simulink library "IP"  (R2014b)
settings: Solver=ode45  StartTime=0.0  StopTime=10.0  RelTol=1e-3
undefined symbols (not defined in the file or in its folder): Serial_Port, Standard_Devices
libraries: IP x7, rtwinlib x4, simulink x2
settings Model: Creator=ZRazer  LastModifiedBy=gt60

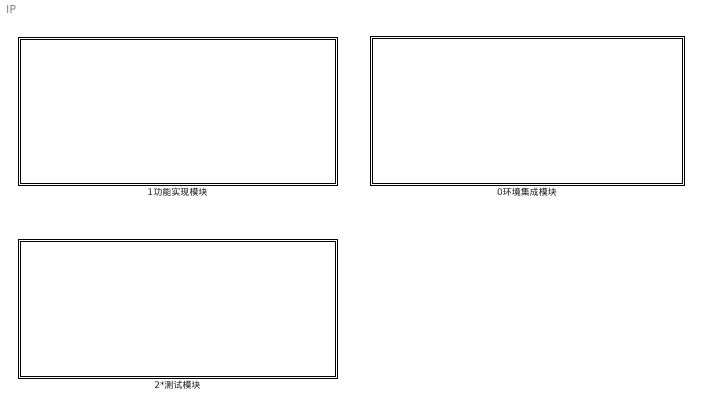
== system IP ==
  0环境集成模块 : Subsystem
  1功能实现模块 : Subsystem
  2*测试模块 : Subsystem

== system IP/0环境集成模块 ==
  倒立摆集成实验 : Subsystem  Description=采样时间dt=0.002s  mask{t=0.002}
      mask prompts: t "sample time(非负数)"
      settings: AttributesFormatString=%<Description>  CopyFcn=set_param(gcbh,'LinkStatus','none');
      mask DialogControl Container5 Prompt: 系统设置
      mask DialogControl ParameterGroupVar Prompt: 采样时间
      mask Display: disp('倒立摆集成模块')
  环境集成实验 : Subsystem  Description=采样时间dt=0.002s  mask{t=0.002}
      mask prompts: t "sample time(非负数)"
      settings: AttributesFormatString=%<Description>  CopyFcn=set_param(gcbh,'LinkStatus','none');
      mask DialogControl Container5 Prompt: 系统设置
      mask DialogControl ParameterGroupVar Prompt: 采样时间
      mask Display: disp('集成环境模块')

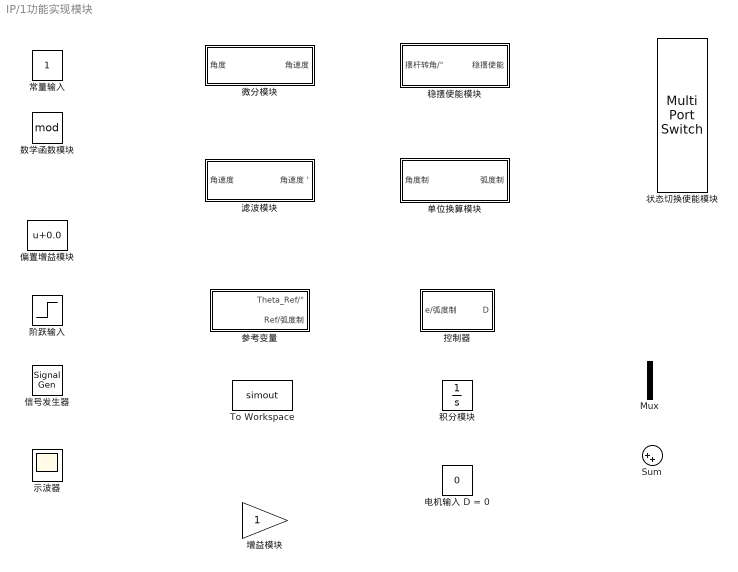
== system IP/1功能实现模块 ==
  Mux : Mux  Inputs=2
  Sum : Sum  Inputs=|++
  To Workspace : ToWorkspace  VariableName=simout  SaveFormat=Timeseries  SampleTime=-1
      settings: AttributesFormatString=%<Description>
      settings: Description=|
      | 数据输出模块
      | 运行完毕后可将连接信号线数据输出到MatLab的工作空间，调用plot命令即可完成数据可视化
      | 调用格式plot(变量名.time，变量名.signals.values)
      | 如：变量名称为theta，在MatLab中调用命令plot(theta.time,theta.signals.values)
  信号发生器 : SignalGenerator  Units=rad/sec
  偏置增益模块 : Bias  Bias=0.0
  单位换算模块 : Subsystem  Description=|
      | 输入：转角(°)或转速(°/s)
      | 输出：转角(rad)或转速(rad/°)
      settings: AttributesFormatString=%<Description>
      mask DialogControl DescGroupVar Prompt: 描述
      mask DialogControl DescTextVar Prompt: 角度制转弧度制
  参考变量 : Subsystem  mask{Amplitude=40, T=10}
      mask prompts: Amplitude "幅值Amplitude/°"; T "周期T/s"
      mask DialogControl Control1 Prompt: 变量期望值
  "增益模块 " : Gain
  常量输入 : Constant
  微分模块 : Subsystem  Description=|
      | 描述：离散微分模块
      | 该部分不必修改
      settings: AttributesFormatString=%<Description>
      mask DialogControl DescGroupVar Prompt: 描述
      mask DialogControl DescTextVar Prompt: 角度-角速度转换
  控制器 : Subsystem  mask{K=[0.0500   0.0258   0.4535   0.0387]}
  数学函数模块 : Math  Description=|  Operator=mod  SaturateOnIntegerOverflow=on
      | 描述：数学函数模块
      | mod 求余函数
      settings: AttributesFormatString=%<Description>
  滤波模块 : Subsystem  Description=|  mask{num=[1], den=[1 2]}
      | 描述：离散滤波模块
      | 先在matlab内构建滤波器的连续传递函数
      | 再内调用c2d()函数
      settings: AttributesFormatString=%<Description>
  状态切换使能模块 : MultiPortSwitch  Description=|  DataPortOrder=Zero-based contiguous  Inputs=2  zeroidx=on
      | 定义左侧端口从上到下分别为输入1~3
      | 输入1：连接稳摆使能端口
      | 输入2：连接常量D=0端口
      | 输入3：连接稳摆控制端口
      | 定义右侧端口为输出端口
      | 输出1：连接控制输入端口
      settings: AttributesFormatString=%<Description>
  "电机输入 D = 0 " : Constant  Description=该模块为输入为0的常量，无法修改  Value=0
      settings: AttributesFormatString=%<Description>
      mask DialogControl DescGroupVar Prompt: 非稳摆状态输入设置
      mask DialogControl DescTextVar Prompt: 控制量u = 0
  示波器 : Scope
      settings: SampleInput=on
  积分模块 : Integrator
  稳摆使能模块 : Subsystem  Description=|  mask{Deg=15}
      | 输入单位：度/°
      | 输出：      0或1
      | 若转角在该范围内，输出1
      | 若转角不在范围内，输出0
      settings: AttributesFormatString=%<Description>
  阶跃输入 : Step  SampleTime=0

== system IP/2*测试模块 ==
  测试模块 : Subsystem  mask{Parameter1=0}

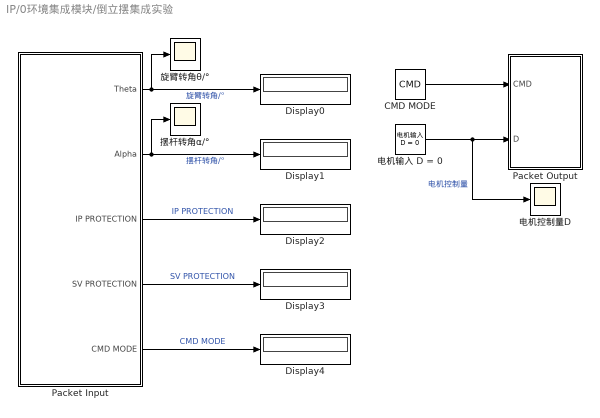
== system IP/0环境集成模块/倒立摆集成实验 ==
  CMD MODE : Constant  Value=CMD  mask{CMD=0}
      mask prompts: CMD "模式选择"
      mask DialogControl DescGroupVar Prompt: 模式切换输入端
      mask DialogControl DescTextVar_copy_copy_copy Prompt: 1:倒立摆模式
      mask DialogControl DescTextVar_copy_copy_copy_copy Prompt: 2:倒立摆异常清除
  Display{0..4} (5 alike) : Display
  Packet Input : Subsystem
  Packet Output : Subsystem
  摆杆转角α/° : Scope
      settings: ShowLegends=on  YMin=-60  YMax=60  SaveName=alpha
  旋臂转角θ/° : Scope
      settings: ShowLegends=on  YMin=-60  YMax=60  SaveName=theta1
  电机控制量D : Scope
      settings: ShowLegends=on  YMin=-0.8  YMax=0.6  SaveName=D
  "电机输入 D = 0 " : IP/附加模块/电机输入 D = 0 
  wires:
  Packet Input/2(Alpha) -> 摆杆转角α/°/1, Display1/1  "摆杆转角/°"
  CMD MODE/1 -> Packet Output/1(CMD)
  Packet Input/1(Theta) -> Display0/1, 旋臂转角θ/°/1  "旋臂转角/°"
  Packet Input/3(IP PROTECTION) -> Display2/1  "IP PROTECTION"
  Packet Input/4(SV PROTECTION) -> Display3/1  "SV PROTECTION"
  Packet Input/5(CMD MODE) -> Display4/1  "CMD MODE"
  "电机输入 D = 0 "/1 -> Packet Output/2(D), 电机控制量D/1  "电机控制量"

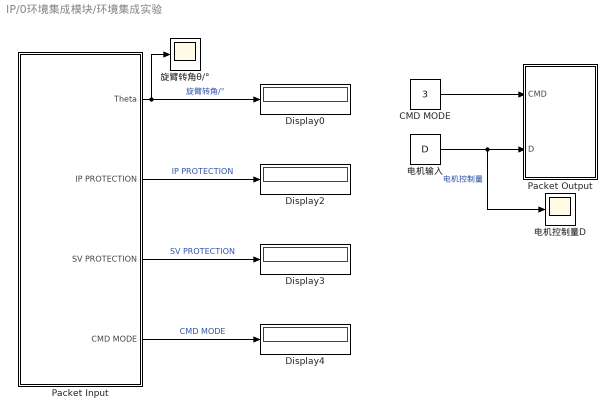
== system IP/0环境集成模块/环境集成实验 ==
  CMD MODE : Constant  Value=3
      mask DialogControl DescGroupVar Prompt: 模式切换输入端
      mask DialogControl DescTextVar Prompt: 当前工作模式：伺服模式(MODE 3）
  Display{0,2..4} (4 alike) : Display
  Packet Input : Subsystem
  Packet Output : Subsystem
  旋臂转角θ/° : Scope
      settings: ShowLegends=on  YMin=-60  YMax=60  SaveName=theta
  电机控制量D : Scope
      settings: ShowLegends=on  YMin=-0.8  YMax=0.6  SaveName=D1
  电机输入 : Constant  Value=D  mask{D=0.0}
      mask DialogControl DescGroupVar Prompt: 电机输入
      mask DialogControl DescTextVar Prompt: 占空比大小
  wires:
  CMD MODE/1 -> Packet Output/1(CMD)
  Packet Input/1(Theta) -> 旋臂转角θ/°/1, Display0/1  "旋臂转角/°"
  Packet Input/2(IP PROTECTION) -> Display2/1  "IP PROTECTION"
  Packet Input/3(SV PROTECTION) -> Display3/1  "SV PROTECTION"
  Packet Input/4(CMD MODE) -> Display4/1  "CMD MODE"
  电机输入/1 -> Packet Output/2(D), 电机控制量D/1  "电机控制量"

== system IP/1功能实现模块/单位换算模块 ==
  角度制 : Inport
  Deg2Rad : Gain  Gain=pi/180
  弧度制 : Outport
  wires:
  角度制/1 -> Deg2Rad/1
  Deg2Rad/1 -> 弧度制/1

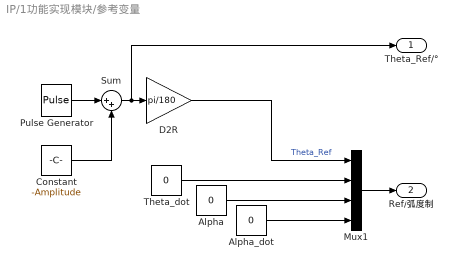
== system IP/1功能实现模块/参考变量 ==
  Alpha : Constant  Value=0
  Alpha_dot : Constant  Value=0
  Constant : Constant  Value=-Amplitude  SampleTime=-1
  D2R : Gain  Gain=pi/180
  Mux1 : Mux
  Pulse Generator : DiscretePulseGenerator  PulseType=Time based  Amplitude=Amplitude*2  Period=T  PulseWidth=50
  Sum : Sum  Inputs=|++
  "Theta_dot " : Constant  Value=0
  Theta_Ref/° : Outport
  Ref/弧度制 : Outport  Port=2
  wires:
  Pulse Generator/1 -> Sum/1
  Constant/1 -> Sum/2
  Sum/1 -> Theta_Ref/°/1, D2R/1
  "Theta_dot "/1 -> Mux1/2
  Alpha_dot/1 -> Mux1/4
  Mux1/1 -> Ref/弧度制/1
  Alpha/1 -> Mux1/3
  D2R/1 -> Mux1/1  "Theta_Ref"

== system IP/1功能实现模块/微分模块 ==
  角度 : Inport
  Difference : simulink/Discrete/Difference  ICPrevInput=0.0  InputProcessing=Inherited  OutMin=[]  OutMax=[]  OutDataType=fixdt(1, 16)  OutScaling=2^-10  DoSatur=off
  补偿1/t : Gain  Gain=1/t
  角速度 : Outport
  wires:
  角度/1 -> Difference/1
  补偿1/t/1 -> 角速度/1
  Difference/1 -> 补偿1/t/1

== system IP/1功能实现模块/控制器 ==
  e/弧度制 : Inport
  Gain : Gain  Gain=K  Multiplication=Matrix(K*u)
  Gain1 : Gain  Gain=-1
  D : Outport
  wires:
  e/弧度制/1 -> Gain/1
  Gain/1 -> Gain1/1
  Gain1/1 -> D/1

== system IP/1功能实现模块/滤波模块 ==
  角速度 : Inport
  Discrete Transfer Fcn1 : DiscreteTransferFcn  Numerator=num  Denominator=den
  角速度 ' : Outport
  wires:
  Discrete Transfer Fcn1/1 -> 角速度 '/1
  角速度/1 -> Discrete Transfer Fcn1/1

== system IP/1功能实现模块/稳摆使能模块 ==
  摆杆转角/° : Inport
  Enable : simulink/Logic and Bit Operations/Compare To Constant  relop=<=  const=Deg  OutDataTypeStr=uint8  ZeroCross=off
  |Alpha_Balance| : Abs
  稳摆使能 : Outport
  wires:
  摆杆转角/°/1 -> |Alpha_Balance|/1
  Enable/1 -> 稳摆使能/1
  |Alpha_Balance|/1 -> Enable/1

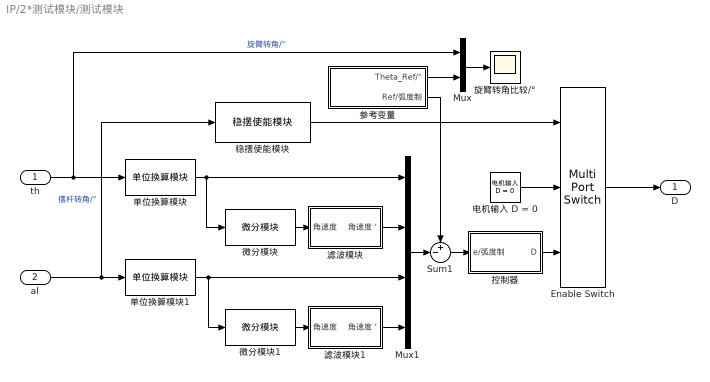
== system IP/2*测试模块/测试模块 ==
  th : Inport
  al : Inport  Port=2
  Enable Switch : MultiPortSwitch  DataPortOrder=Zero-based contiguous  Inputs=2  zeroidx=on
  Mux : Mux  Inputs=2
  Mux1 : Mux
  Sum1 : Sum  Inputs=+-|
  单位换算模块 : IP/附加模块/单位换算模块
      settings: AttributesFormatString=%<Description>
  单位换算模块1 : IP/附加模块/单位换算模块
      settings: AttributesFormatString=%<Description>
  参考变量 : Subsystem  mask{Amplitude=40, T=10}
      mask prompts: Amplitude "幅值Amplitude/°"; T "周期T/s"
      mask DialogControl Control1 Prompt: 变量期望值
  微分模块 : IP/附加模块/微分模块
      settings: AttributesFormatString=%<Description>
  微分模块1 : IP/附加模块/微分模块
      settings: AttributesFormatString=%<Description>
  控制器 : Subsystem  mask{K=[0.0500   0.0258   0.4535   0.0387]}
  旋臂转角比较/° : Scope
      settings: ShowLegends=on  YMin=-80  YMax=80  SaveName=cmp
  滤波模块 : Subsystem  mask{num=[0.2212], den=[1 -0.7788]}
      settings: AttributesFormatString=%<Description>
  滤波模块1 : Subsystem  mask{num=[0.2212], den=[1 -0.7788]}
      settings: AttributesFormatString=%<Description>
  "电机输入 D = 0 " : IP/附加模块/电机输入 D = 0 
  稳摆使能模块 : IP/附加模块/稳摆使能模块  Deg=15
      settings: AttributesFormatString=%<Description>
  D : Outport
  wires:
  al/1 -> 稳摆使能模块/1, 单位换算模块1/1  "摆杆转角/°"
  th/1 -> Mux/1, 单位换算模块/1  "旋臂转角/°"
  "电机输入 D = 0 "/1 -> Enable Switch/2
  稳摆使能模块/1 -> Enable Switch/1
  单位换算模块1/1 -> 微分模块1/1, Mux1/3
  微分模块/1 -> 滤波模块/1(角速度)
  微分模块1/1 -> 滤波模块1/1(角速度)
  滤波模块/1(角速度 ') -> Mux1/2
  滤波模块1/1(角速度 ') -> Mux1/4
  参考变量/1(Theta_Ref/°) -> Mux/2
  Mux/1 -> 旋臂转角比较/°/1
  单位换算模块/1 -> 微分模块/1, Mux1/1
  Sum1/1 -> 控制器/1(e/弧度制)
  Mux1/1 -> Sum1/2
  参考变量/2(Ref/弧度制) -> Sum1/1
  控制器/1(D) -> Enable Switch/3
  Enable Switch/1 -> D/1

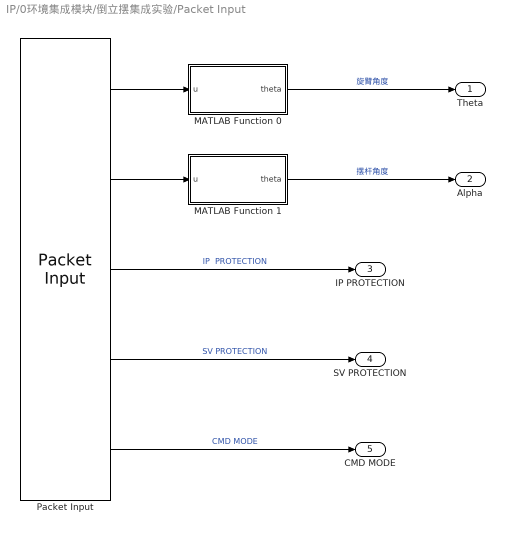
== system IP/0环境集成模块/倒立摆集成实验/Packet Input ==
  MATLAB Function 0 : MATLAB Function  TreatAsAtomicUnit=on
  MATLAB Function 1 : MATLAB Function  TreatAsAtomicUnit=on
  Packet Input : rtwinlib/Packet Input  SampleTime=t  MaxMissedTicks=10  ShowMissedTicks=off  YieldWhenWaiting=off  DrvName=Standard_Devices/Serial_Port  DrvAddress=3  DrvOptions=[460800 8 0 0 0 0 0 0]  PacketSize=9  DataTypes={'int32','int16','uint8','uint8','uint8'}  ShowReady=off  ShowError=off  PacketID=1  ByteOrder=1  ShowTimestamp=off
      settings: AttributesFormatString=Standard Devices\nSerial Port [3h]
  Theta : Outport
  Alpha : Outport  Port=2
  IP PROTECTION : Outport  Port=3
  SV PROTECTION : Outport  Port=4
  CMD MODE : Outport  Port=5
  wires:
  MATLAB Function 1/1(theta) -> Alpha/1  "摆杆角度"
  Packet Input/5 -> CMD MODE/1  "CMD MODE"
  Packet Input/3 -> IP PROTECTION/1  "IP  PROTECTION"
  Packet Input/4 -> SV PROTECTION/1  "SV PROTECTION"
  Packet Input/2 -> MATLAB Function 1/1(u)
  Packet Input/1 -> MATLAB Function 0/1(u)
  MATLAB Function 0/1(theta) -> Theta/1  "旋臂角度"

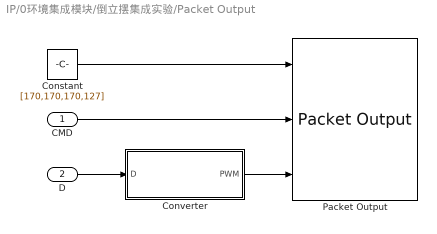
== system IP/0环境集成模块/倒立摆集成实验/Packet Output ==
  CMD : Inport
  D : Inport  Port=2
  Constant : Constant  Value=[170,170,170,127]
      mask DialogControl DescGroupVar Prompt: 描述
      mask DialogControl DescTextVar Prompt: 常量
  Converter : Subsystem  mask{k=0.3}
      mask DialogControl DescTextVar Prompt: 数学变换
  Packet Output : rtwinlib/Packet Output  SampleTime=t  MaxMissedTicks=10  ShowMissedTicks=off  YieldWhenWaiting=off  DrvName=Standard_Devices/Serial_Port  DrvAddress=3  DrvOptions=[460800 8 0 0 0 0 0 0]  PacketSize=7  DataTypes={'4*uint8','uint8','int16'}  ShowReady=off  ShowError=off  PacketID=1  ByteOrder=1  InitialValue=[170 170 170 127 1 0]  FinalValue=[]
      settings: AttributesFormatString=Standard Devices\nSerial Port [3h]
  wires:
  D/1 -> Converter/1(D)
  Constant/1 -> Packet Output/1
  Converter/1(PWM) -> Packet Output/3
  CMD/1 -> Packet Output/2

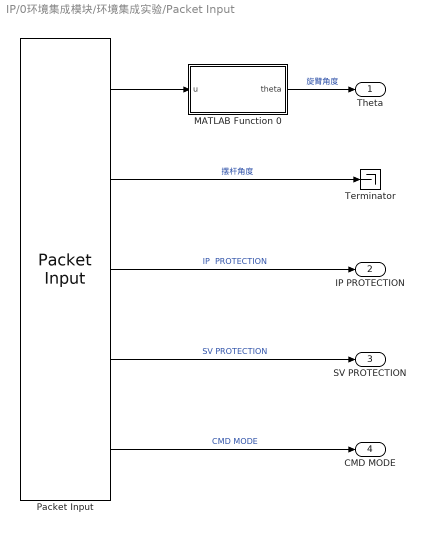
== system IP/0环境集成模块/环境集成实验/Packet Input ==
  MATLAB Function 0 : MATLAB Function  TreatAsAtomicUnit=on
  Packet Input : rtwinlib/Packet Input  SampleTime=t  MaxMissedTicks=10  ShowMissedTicks=off  YieldWhenWaiting=off  DrvName=Standard_Devices/Serial_Port  DrvAddress=3  DrvOptions=[460800 8 0 0 0 0 0 0]  PacketSize=9  DataTypes={'int32','int16','uint8','uint8','uint8'}  ShowReady=off  ShowError=off  PacketID=1  ByteOrder=1  ShowTimestamp=off
      settings: AttributesFormatString=Standard Devices\nSerial Port [3h]
  Terminator : Terminator
  Theta : Outport
  IP PROTECTION : Outport  Port=2
  SV PROTECTION : Outport  Port=3
  CMD MODE : Outport  Port=4
  wires:
  Packet Input/2 -> Terminator/1  "摆杆角度"
  Packet Input/5 -> CMD MODE/1  "CMD MODE"
  Packet Input/3 -> IP PROTECTION/1  "IP  PROTECTION"
  Packet Input/4 -> SV PROTECTION/1  "SV PROTECTION"
  Packet Input/1 -> MATLAB Function 0/1(u)
  MATLAB Function 0/1(theta) -> Theta/1  "旋臂角度"

== system IP/0环境集成模块/环境集成实验/Packet Output ==
  CMD : Inport
  D : Inport  Port=2
  Constant : Constant  Value=[170,170,170,127]
      mask DialogControl DescGroupVar Prompt: 描述
      mask DialogControl DescTextVar Prompt: 常量
  Converter : Subsystem  mask{k=0.3}
      mask DialogControl DescTextVar Prompt: 数学变换
  Packet Output : rtwinlib/Packet Output  SampleTime=t  MaxMissedTicks=10  ShowMissedTicks=off  YieldWhenWaiting=off  DrvName=Standard_Devices/Serial_Port  DrvAddress=3  DrvOptions=[460800 8 0 0 0 0 0 0]  PacketSize=7  DataTypes={'4*uint8','uint8','int16'}  ShowReady=off  ShowError=off  PacketID=1  ByteOrder=1  InitialValue=[170 170 170 127 1 0]  FinalValue=[]
      settings: AttributesFormatString=Standard Devices\nSerial Port [3h]
  wires:
  CMD/1 -> Packet Output/2
  Converter/1(PWM) -> Packet Output/3
  Constant/1 -> Packet Output/1
  D/1 -> Converter/1(D)

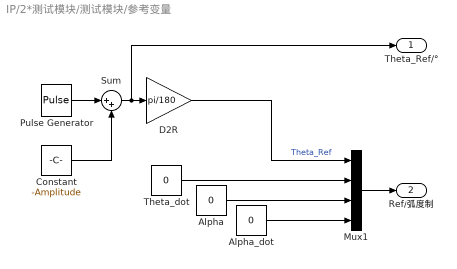
== system IP/2*测试模块/测试模块/参考变量 ==
  Alpha : Constant  Value=0
  Alpha_dot : Constant  Value=0
  Constant : Constant  Value=-Amplitude
  D2R : Gain  Gain=pi/180
  Mux1 : Mux
  Pulse Generator : DiscretePulseGenerator  PulseType=Time based  Amplitude=Amplitude*2  Period=T  PulseWidth=50
  Sum : Sum  Inputs=|++
  "Theta_dot " : Constant  Value=0
  Theta_Ref/° : Outport
  Ref/弧度制 : Outport  Port=2
  wires:
  Pulse Generator/1 -> Sum/1
  Constant/1 -> Sum/2
  Sum/1 -> Theta_Ref/°/1, D2R/1
  "Theta_dot "/1 -> Mux1/2
  Alpha_dot/1 -> Mux1/4
  Mux1/1 -> Ref/弧度制/1
  Alpha/1 -> Mux1/3
  D2R/1 -> Mux1/1  "Theta_Ref"

== system IP/2*测试模块/测试模块/控制器 ==
  e/弧度制 : Inport
  Gain : Gain  Gain=K  Multiplication=Matrix(K*u)
  Gain1 : Gain  Gain=-1
  D : Outport
  wires:
  e/弧度制/1 -> Gain/1
  Gain/1 -> Gain1/1
  Gain1/1 -> D/1

== system IP/2*测试模块/测试模块/滤波模块 ==
  角速度 : Inport
  Discrete Transfer Fcn1 : DiscreteTransferFcn  Numerator=num  Denominator=den
  角速度 ' : Outport
  wires:
  角速度/1 -> Discrete Transfer Fcn1/1
  Discrete Transfer Fcn1/1 -> 角速度 '/1

== system IP/2*测试模块/测试模块/滤波模块1 ==
  角速度 : Inport
  Discrete Transfer Fcn1 : DiscreteTransferFcn  Numerator=num  Denominator=den
  角速度 ' : Outport
  wires:
  Discrete Transfer Fcn1/1 -> 角速度 '/1
  角速度/1 -> Discrete Transfer Fcn1/1

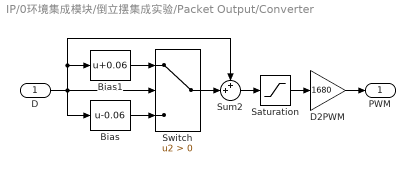
== system IP/0环境集成模块/倒立摆集成实验/Packet Output/Converter ==
  D : Inport
  Bias : Bias  Bias=-0.06
  Bias1 : Bias  Bias=0.06
  D2PWM : Gain  Gain=1680
      mask DialogControl Container4 Prompt: 描述
      mask DialogControl DescTextVar Prompt: 输入占空比-输入PWM
  Saturation : Saturate  UpperLimit=k  LowerLimit=-k
  Sum2 : Sum  Inputs=++|
  Switch : Switch  Criteria=u2 > Threshold
  PWM : Outport
  wires:
  D2PWM/1 -> PWM/1
  Saturation/1 -> D2PWM/1
  D/1 -> Bias/1, Switch/2, Sum2/1, Bias1/1
  Bias/1 -> Switch/3
  Bias1/1 -> Switch/1
  Switch/1 -> Sum2/2
  Sum2/1 -> Saturation/1

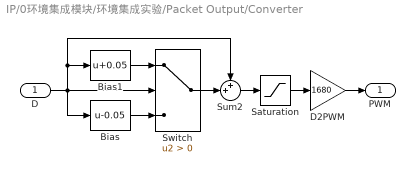
== system IP/0环境集成模块/环境集成实验/Packet Output/Converter ==
  D : Inport
  Bias : Bias  Bias=-0.05
  Bias1 : Bias  Bias=0.05
  D2PWM : Gain  Gain=1680
      mask DialogControl Container4 Prompt: 描述
      mask DialogControl DescTextVar Prompt: 输入占空比-输入PWM
  Saturation : Saturate  UpperLimit=k  LowerLimit=-k
  Sum2 : Sum  Inputs=++|
  Switch : Switch  Criteria=u2 > Threshold
  PWM : Outport
  wires:
  Sum2/1 -> Saturation/1
  Switch/1 -> Sum2/2
  Bias1/1 -> Switch/1
  Bias/1 -> Switch/3
  D/1 -> Bias1/1, Sum2/1, Switch/2, Bias/1
  Saturation/1 -> D2PWM/1
  D2PWM/1 -> PWM/1

== matlab function IP/0环境集成模块/环境集成实验/Packet Input/MATLAB Function 0 ==
  data: u input; theta output
function theta = fcn(u)
%函数输入输出定义如下：
%输入u    ：编码器旋转码数（单位：码）
%输出theta：转轴旋转角度（单位：°）
%=====不要修改下方代码块=====%
    u = double(u);
%=====不要修改上方代码块=====%

%例：
%   有一512码/圈编码器，倍频数2，减速机倍频14
%   旋转一圈  360°对应512*2*14码
%   theta = u*360/512/2/14；
%   该处编码器500/圈，倍频数4，减速器倍频25
%=======下方输入代码=======%
    theta=u*360/1/1/1;
%=======上方输入代码=======%
end

== matlab function IP/0环境集成模块/倒立摆集成实验/Packet Input/MATLAB Function 0 ==
  data: u input; theta output
function theta = fcn(u)
%函数输入输出定义如下：
%输入u    ：编码器旋转码数（单位：码）
%输出theta：转轴旋转角度（单位：°）
%=====不要修改下方代码块=====%
    u = double(u);
%=====不要修改上方代码块=====%

%例：
%   有一512码/圈编码器，倍频数2，减速机倍频14
%   旋转一圈  360°对应512*2*14码
%   theta = u*360/512/2/14；
%   该处编码器500/圈，倍频数4，减速器倍频25
%=======下方输入代码=======%
    theta=u*360/1/1/1;
%=======上方输入代码=======%
end

== matlab function IP/0环境集成模块/倒立摆集成实验/Packet Input/MATLAB Function 1 ==
  data: u input; theta output
function theta = fcn(u)
%函数输入输出定义如下：
%输入u    ：编码器旋转码数（单位：码）
%输出theta：转轴旋转角度（单位：°）
%=====不要修改下方代码块=====%
if(u>=2^15)
    %negative number
    u = u - 2^16;
end
    u = double(u);
%=====不要修改上方代码块=====%

%例：
%   有一512码/圈编码器，倍频数2，减速机倍频14
%   旋转一圈  360°对应512*2*14码
%   theta = u*360/512/2/14；
%   该处编码器1024/圈，倍频数4，无减速器倍频
%=======下方输入代码=======%
    theta=u*360/1/1;
%=======上方输入代码=======%
end
